simulink model "signal"  (R2015a)
settings: Solver=ode45  StartTime=0.0  StopTime=0.02  RelTol=1e-3
libraries: powerlib x14, simulink x4
settings Model: Creator=User  LastModifiedBy=User

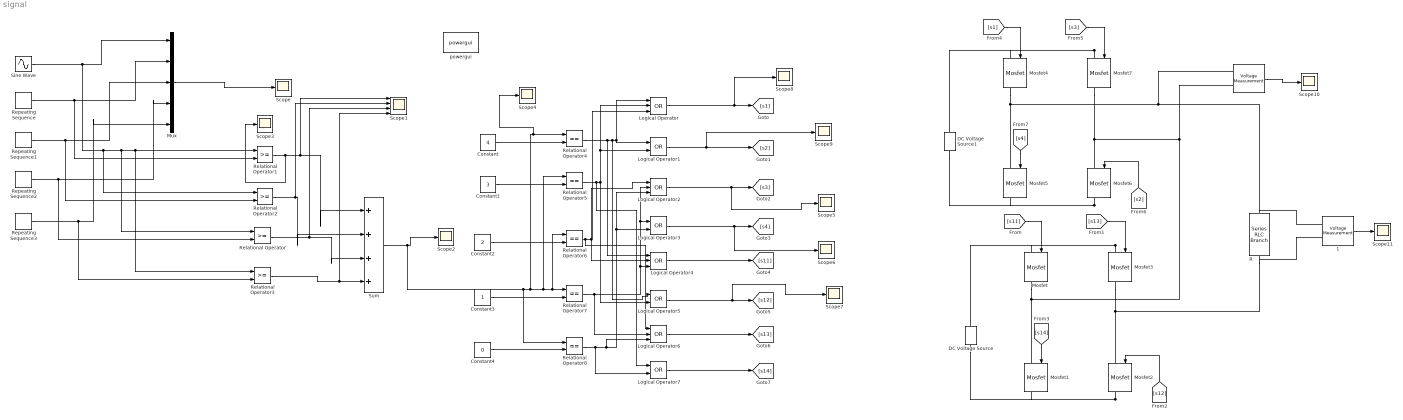
== system signal ==
  " " : powerlib/Measurements/Voltage Measurement  PhasorSimulation=off  OutputType=Complex  PSBequivalent=0
  " 1" : powerlib/Measurements/Voltage Measurement  PhasorSimulation=off  OutputType=Complex  PSBequivalent=0
  Constant : Constant  Value=4
  Constant1 : Constant  Value=3
  Constant2 : Constant  Value=2
  Constant3 : Constant
  Constant4 : Constant  Value=0
  DC Voltage Source : powerlib/Electrical Sources/DC Voltage Source  Amplitude=400  Measurements=None
  DC Voltage Source1 : powerlib/Electrical Sources/DC Voltage Source  Amplitude=400  Measurements=None
  Logical Operator{,2,4,6} (4 alike) : Logic  Operator=OR  Inputs=3  AllPortsSameDT=off  OutDataTypeStr=boolean
  Logical Operator{1,3,5,7} (4 alike) : Logic  Operator=OR  AllPortsSameDT=off  OutDataTypeStr=boolean
  Mosfet{,1..7} (8 alike) : powerlib/Power Electronics/Mosfet  Ron=0.1  Lon=0  Rd=0.01  Vfd=0  IC=0  Rs=1e5  Cs=inf  Measurements=on
  Mux : Mux  Inputs=5
  R : powerlib/Elements/Series RLC Branch  LConnTagsString=__new0  RConnTagsString=__new0  BranchType=R  Resistance=100  Inductance=1e-3  SetiL0=off  InitialCurrent=0  Capacitance=1e-6  Setx0=off  InitialVoltage=0  Measurements=Branch voltage
  Relational Operator{,1..3} (4 alike) : RelationalOperator  OutDataTypeStr=boolean
  Relational Operator{4..8} (5 alike) : RelationalOperator  Operator===  OutDataTypeStr=boolean
  Repeating Sequence : simulink/Sources/Repeating Sequence  rep_seq_t=[0 1 2]*[1/400]  rep_seq_y=[1 2 1]
  Repeating Sequence1 : simulink/Sources/Repeating Sequence  rep_seq_t=[0 1 2]*[1/400]  rep_seq_y=[0 1 0]
  Repeating Sequence2 : simulink/Sources/Repeating Sequence  rep_seq_t=[0 1 2]*[1/400]  rep_seq_y=[0 -1 0]
  Repeating Sequence3 : simulink/Sources/Repeating Sequence  rep_seq_t=[0 1 2]*[1/400]  rep_seq_y=[-1 -2 -1 ]
  Scope{,2..11} (11 alike) : Scope
      Scope10 settings: SaveName=ScopeData10
      Scope11 settings: SaveName=ScopeData11
      Scope2 settings: SaveName=ScopeData2
      Scope3 settings: SaveName=ScopeData3
      Scope4 settings: SaveName=ScopeData4
      Scope5 settings: SaveName=ScopeData5
      Scope6 settings: SaveName=ScopeData6
      Scope7 settings: SaveName=ScopeData7
      Scope8 settings: SaveName=ScopeData8
      Scope9 settings: SaveName=ScopeData9
  Scope1 : Scope  NumInputPorts=4
      settings: TimeRange=0.02  YMin=-5~-5~-5~-5  YMax=5~5~5~5
  Sine Wave : Sin  Amplitude=2  Frequency=2*pi*50  SampleTime=0
  Sum : Sum  Inputs=|++++
  powergui : powerlib/powergui  Priority=1  SimulationMode=Continuous  SolverType=Tustin/Backward Euler (TBE)  SampleTime=50e-6  frequency=60  SPID=off  DisableSnubberDevices=off  DisableRonSwitches=off  DisableVfSwitches=off  SwTol=0  DisplayEquations=off  Interpol=off  methode=off  Ts=100  FunctionMessages=off  echomessages=off  HookPort=off  EnableUseOfTLC=off  x0status=blocks  frequencyindice=0  Pbase=100e6  ErrMax=1e-4  Iterations=50  UnitsV=kV  UnitsW=MW  buscounter=0  RestoreLinks=warning  ResistiveCurrentMeasurement=off  Frange=[0:2:500]  Ylog=off  Xlog=on  ShowGrid=off  save=off  variable=ZData  structure=0  ZoomFFT=off  StartTime=0.0  cycles=1  DisplayStyle=1  fundamental=60  FreqAxis=off  MaxFrequency=1000  frequencyindicesteady=1  RmsSteady=1  display=off
  wires:
  Sine Wave/1 -> Relational Operator2/1, Relational Operator/1, Relational Operator3/1, Relational Operator1/1, Mux/1
  Repeating Sequence/1 -> Relational Operator1/2, Mux/2
  Repeating Sequence1/1 -> Relational Operator2/2, Mux/3
  Repeating Sequence2/1 -> Relational Operator/2, Mux/4
  Repeating Sequence3/1 -> Relational Operator3/2, Mux/5
  Mux/1 -> Scope/1
  Relational Operator1/1 -> Scope3/1, Scope1/1, Sum/1
  Relational Operator2/1 -> Scope1/2, Sum/2
  Relational Operator/1 -> Scope1/3, Sum/3
  Relational Operator3/1 -> Scope1/4, Sum/4
  Sum/1 -> Relational Operator8/1, Scope4/1, Relational Operator4/1, Relational Operator5/1, Relational Operator6/1, Relational Operator7/1, Scope2/1
  Constant4/1 -> Relational Operator8/2
  Constant3/1 -> Relational Operator7/2
  Constant2/1 -> Relational Operator6/2
  Constant1/1 -> Relational Operator5/2
  Constant/1 -> Relational Operator4/2
  Relational Operator4/1 -> Logical Operator4/1, Logical Operator5/1, Logical Operator/1, Logical Operator1/1
  Relational Operator5/1 -> Logical Operator7/1, Logical Operator1/2, Logical Operator/2, Logical Operator5/2
  Relational Operator6/1 -> Logical Operator6/1, Logical Operator4/2, Logical Operator2/1, Logical Operator/3
  Relational Operator7/1 -> Logical Operator6/2, Logical Operator4/3, Logical Operator3/1, Logical Operator2/2
  Relational Operator8/1 -> Logical Operator7/2, Logical Operator6/3, Logical Operator3/2, Logical Operator2/3
  Logical Operator/1 -> Scope8/1, [s1]
  Logical Operator1/1 -> Scope9/1, [s2]
  Logical Operator2/1 -> Scope5/1, [s3]
  Logical Operator3/1 -> Scope6/1, [s4]
  Logical Operator4/1 -> [s11]
  Logical Operator6/1 -> [s13]
  Logical Operator7/1 -> [s14]
  Logical Operator5/1 -> Scope7/1, [s12]
  [s11] -> Mosfet/1
  [s12] -> Mosfet2/1
  [s13] -> Mosfet3/1
  [s14] -> Mosfet1/1
  [s1] -> Mosfet4/1
  [s2] -> Mosfet6/1
  [s3] -> Mosfet7/1
  [s4] -> Mosfet5/1
  " "/1 -> Scope10/1
  " 1"/1 -> Scope11/1
  connections:
  Mosfet3/LConn1 -- DC Voltage Source/RConn1 -- Mosfet/LConn1
  Mosfet2/RConn1 -- DC Voltage Source/LConn1 -- Mosfet1/RConn1
  Mosfet3/RConn1 -- " 1"/LConn2 -- R/RConn1 -- Mosfet2/LConn1
  Mosfet7/LConn1 -- DC Voltage Source1/RConn1 -- Mosfet4/LConn1
  Mosfet6/RConn1 -- DC Voltage Source1/LConn1 -- Mosfet5/RConn1
  Mosfet4/RConn1 -- " 1"/LConn1 -- R/LConn1 -- " "/LConn1 -- Mosfet5/LConn1
  Mosfet/RConn1 -- " "/LConn2 -- Mosfet6/LConn1 -- Mosfet7/RConn1 -- Mosfet1/LConn1
